simulink model "CarClosedLoopLine"  (Simulink 7.7)
settings: Solver=ode45  StartTime=0.0  StopTime=60.0  RelTol=1e-3
values from neighbouring files (symbols this model uses):
  den = ctr.den{1}    [car1.m]    (also in car2.m; car3.m; car4.m; pendulum.m)
  L = 0.2    [car1.m]    (also in car2.m; car3.m; car4.m)
  num = ctr.num{1}    [car1.m]    (also in car2.m; car3.m; car4.m; pendulum.m = K * ctr.num{1})
  RyBar = 1    [car1.m]    (also in car2.m = 10; car3.m; car4.m)
  v = 1    [car1.m]    (also in car2.m; car3.m = -1; car4.m)
settings Model: Creator=mauricio  LastModifiedBy=mauricio
settings DebuggingCC: SolverPrmCheckMsg=none

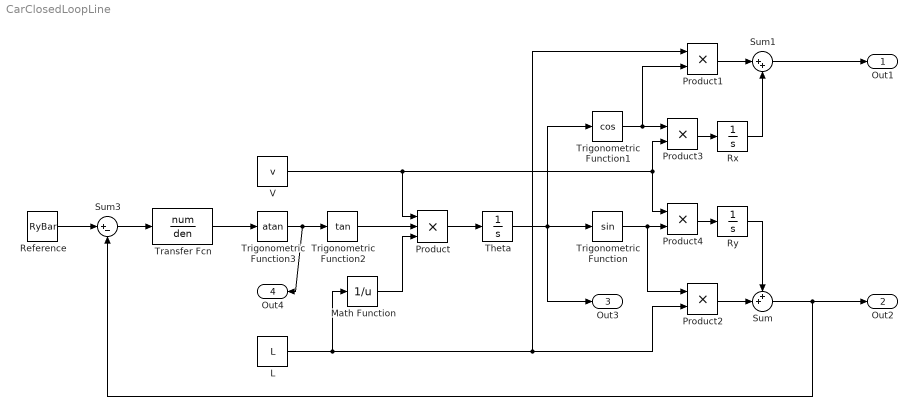
== system CarClosedLoopLine ==
  L : Constant  Value=L
  Math Function : Math  Operator=reciprocal  SaturateOnIntegerOverflow=on
  Product : Product  Inputs=3  RndMeth=Zero
  Product{1..4} (4 alike) : Product  RndMeth=Zero
  Reference : Constant  Value=RyBar
  Rx : Integrator
  Ry : Integrator
  Sum : Sum  Inputs=++|
  Sum1 : Sum  Inputs=|++
  Sum3 : Sum  Inputs=|+-
  Theta : Integrator
  Transfer Fcn : TransferFcn  Numerator=num  Denominator=den
  Trigonometric Function : Trigonometry
  Trigonometric Function1 : Trigonometry  Operator=cos
  Trigonometric Function2 : Trigonometry  Operator=tan
  Trigonometric Function3 : Trigonometry  Operator=atan
  V : Constant  Value=v
  Out1 : Outport
  Out2 : Outport  Port=2
  Out3 : Outport  Port=3
  Out4 : Outport  Port=4
  wires:
  Trigonometric Function1/1 -> Product1/2, Product3/1
  Trigonometric Function/1 -> Product2/1, Product4/2
  Theta/1 -> Trigonometric Function/1, Trigonometric Function1/1, Out3/1
  Product/1 -> Theta/1
  Rx/1 -> Sum1/2
  Ry/1 -> Sum/1
  L/1 -> Math Function/1, Product2/2, Product1/1
  Product1/1 -> Sum1/1
  Product2/1 -> Sum/2
  Sum1/1 -> Out1/1
  Sum/1 -> Out2/1, Sum3/2
  Product4/1 -> Ry/1
  Product3/1 -> Rx/1
  V/1 -> Product3/2, Product4/1, Product/1
  Trigonometric Function2/1 -> Product/2
  Math Function/1 -> Product/3
  Transfer Fcn/1 -> Trigonometric Function3/1
  Trigonometric Function3/1 -> Trigonometric Function2/1, Out4/1
  Reference/1 -> Sum3/1
  Sum3/1 -> Transfer Fcn/1
